simulink model "InverseDynamicsControlOperational"  (R2021b)
settings: Solver=VariableStepAuto  StartTime=0.0  StopTime=15  RelTol=1e-3
values from neighbouring files (symbols this model uses):
  F_v = zeros(6,6)    [param.m]
  K_d = 200.*eye(6,6)    [param.m]
  K_p = 1000.*eye(6,6)    [param.m]
undefined symbols (not defined in the file or in its folder): a, g, iner_l, pi_l, q_i
settings Model: Creator=ASUS  LastModifiedBy=ASUS

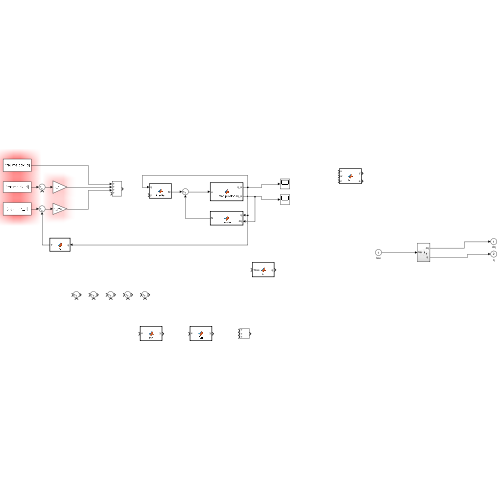
[thumbnail: Simulink's stored preview of the top-level diagram]
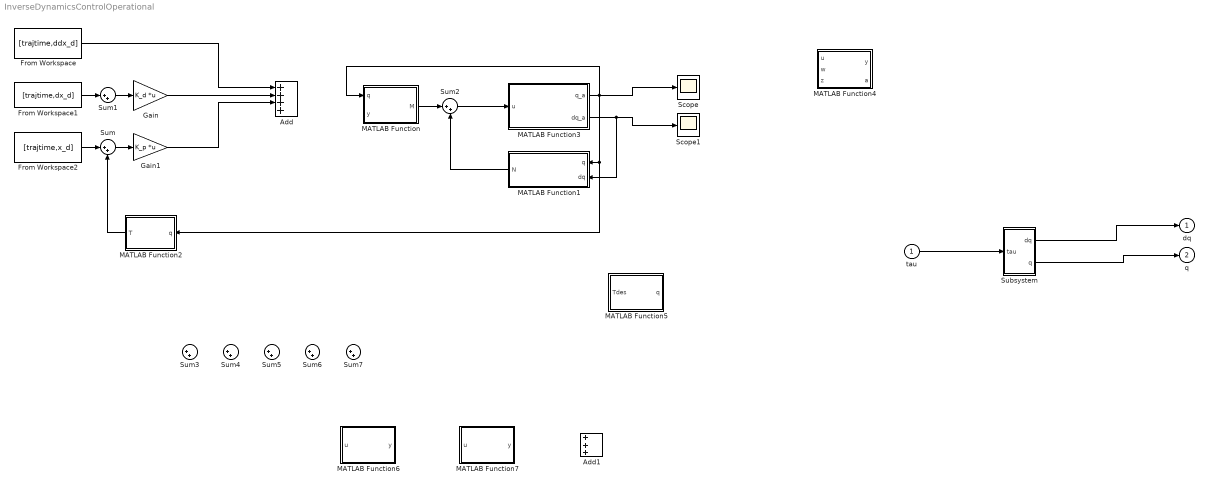
== system InverseDynamicsControlOperational ==
  tau : Inport
  Add : Sum  Inputs=++++
  Add1 : Sum  Inputs=+++
  From Workspace : FromWorkspace  VariableName=[trajtime,ddx_d]
  From Workspace1 : FromWorkspace  VariableName=[trajtime,dx_d]
  From Workspace2 : FromWorkspace  VariableName=[trajtime,x_d]
  Gain : Gain  Gain=K_d  Multiplication=Matrix(K*u)
  Gain1 : Gain  Gain=K_p  Multiplication=Matrix(K*u)
  MATLAB Function : MATLAB Function  TreatAsAtomicUnit=on
  MATLAB Function1 : MATLAB Function  TreatAsAtomicUnit=on
  MATLAB Function2 : MATLAB Function  TreatAsAtomicUnit=on
  MATLAB Function3 : MATLAB Function  TreatAsAtomicUnit=on
  MATLAB Function4 : MATLAB Function  TreatAsAtomicUnit=on
  MATLAB Function5 : MATLAB Function  TreatAsAtomicUnit=on
  MATLAB Function6 : MATLAB Function  TreatAsAtomicUnit=on
  MATLAB Function7 : MATLAB Function  TreatAsAtomicUnit=on
  Scope : Scope
  Scope1 : Scope
  Subsystem : Subsystem
  Sum{,1..7} (8 alike) : Sum  Inputs=|++
  dq : Outport  InitialOutput=0
  "q " : Outport  Port=2  InitialOutput=0
  wires:
  From Workspace/1 -> Add/1
  Gain/1 -> Add/2
  Gain1/1 -> Add/3
  From Workspace2/1 -> Sum/1
  Sum/1 -> Gain1/1
  From Workspace1/1 -> Sum1/1
  Sum1/1 -> Gain/1
  MATLAB Function2/1(T) -> Sum/2
  MATLAB Function/1(M) -> Sum2/1
  MATLAB Function1/1(N) -> Sum2/2
  Sum2/1 -> MATLAB Function3/1(u)
  MATLAB Function3/1(q_a) -> MATLAB Function/1(q), Scope/1, MATLAB Function2/1(q), MATLAB Function1/1(q)
  MATLAB Function3/2(dq_a) -> MATLAB Function1/2(dq), Scope1/1
  tau/1 -> Subsystem/1(tau)
  Subsystem/1(dq) -> dq/1
  Subsystem/2("q ") -> "q "/1

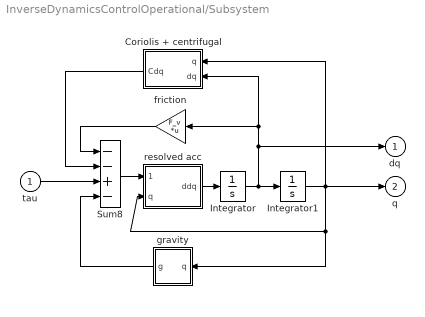
== system InverseDynamicsControlOperational/Subsystem ==
  tau : Inport
  Coriolis + centrifugal : Subsystem
      mask Display: disp('C(q,dq)dq')
  Integrator : Integrator  InitialCondition=[0 0]  ZeroCross=off
  Integrator1 : Integrator  InitialCondition=q_i  ZeroCross=off
  Sum8 : Sum  Inputs=--+-  InputSameDT=on  SaturateOnIntegerOverflow=on  OutDataTypeStr=Inherit: Same as first input
  friction : Gain  Gain=F_v  Multiplication=Matrix(K*u)  SaturateOnIntegerOverflow=on  OutDataTypeStr=Inherit: Same as input  ParamDataTypeStr=Inherit: Same as input
      mask Display: disp('F_v')
  gravity : Subsystem
      mask Display: disp('g(q)')
  resolved acc : Subsystem
      mask Display: disp('inv(B(q))')
  dq : Outport  InitialOutput=0
  "q " : Outport  Port=2  InitialOutput=0
  wires:
  Integrator/1 -> Integrator1/1, dq/1, Coriolis + centrifugal/2(dq), friction/1
  Integrator1/1 -> "q "/1, Coriolis + centrifugal/1(q), resolved acc/2(q), gravity/1(q)
  Sum8/1 -> resolved acc/1(tau-tau')
  gravity/1(g) -> Sum8/4
  tau/1 -> Sum8/3
  Coriolis + centrifugal/1(Cdq) -> Sum8/2
  friction/1 -> Sum8/1
  resolved acc/1(ddq) -> Integrator/1

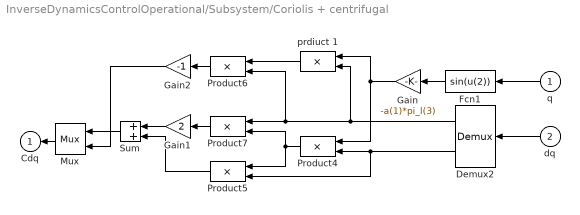
== system InverseDynamicsControlOperational/Subsystem/Coriolis + centrifugal ==
  q : Inport
  dq : Inport  Port=2
  Demux2 : Demux  Outputs=2
      settings: DisplayOption=none
  Fcn1 : Fcn  Expr=sin(u(2))
  Gain : Gain  Gain=-a(1)*pi_l(3)  SaturateOnIntegerOverflow=on  OutDataTypeStr=Inherit: Same as input  ParamDataTypeStr=Inherit: Same as input
      mask Display: disp('k_3')
  Gain1 : Gain  Gain=2  SaturateOnIntegerOverflow=on  OutDataTypeStr=Inherit: Same as input  ParamDataTypeStr=Inherit: Same as input
  Gain2 : Gain  Gain=-1  SaturateOnIntegerOverflow=on  OutDataTypeStr=Inherit: Same as input  ParamDataTypeStr=Inherit: Same as input
  Mux : Mux  Inputs=2
  Product{4..7} (4 alike) : Product  InputSameDT=on  RndMeth=Zero  SaturateOnIntegerOverflow=on  OutDataTypeStr=Inherit: Same as first input
  Sum : Sum  InputSameDT=on  SaturateOnIntegerOverflow=on  OutDataTypeStr=Inherit: Same as first input
  prdiuct 1 : Product  InputSameDT=on  RndMeth=Zero  SaturateOnIntegerOverflow=on  OutDataTypeStr=Inherit: Same as first input
  Cdq : Outport  InitialOutput=0
  wires:
  dq/1 -> Demux2/1
  Gain2/1 -> Mux/2
  Product6/1 -> Gain2/1
  Mux/1 -> Cdq/1
  Sum/1 -> Mux/1
  Product5/1 -> Sum/2
  Gain1/1 -> Sum/1
  Product7/1 -> Gain1/1
  Demux2/1 -> prdiuct 1/2, Product6/2, Product7/1
  Demux2/2 -> Product4/2, Product5/2
  prdiuct 1/1 -> Product6/1
  Gain/1 -> prdiuct 1/1, Product4/1
  Fcn1/1 -> Gain/1
  q/1 -> Fcn1/1
  Product4/1 -> Product5/1, Product7/2

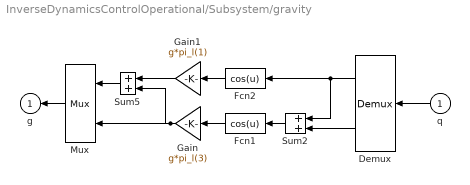
== system InverseDynamicsControlOperational/Subsystem/gravity ==
  q : Inport
  Demux : Demux  Outputs=2
      settings: DisplayOption=none
  Fcn1 : Fcn  Expr=cos(u)
  Fcn2 : Fcn  Expr=cos(u)
  Gain : Gain  Gain=g*pi_l(3)  SaturateOnIntegerOverflow=on  OutDataTypeStr=Inherit: Same as input  ParamDataTypeStr=Inherit: Same as input
      mask Display: disp('k_2')
  Gain1 : Gain  Gain=g*pi_l(1)  SaturateOnIntegerOverflow=on  OutDataTypeStr=Inherit: Same as input  ParamDataTypeStr=Inherit: Same as input
      mask Display: disp('k_1')
  Mux : Mux  Inputs=2
  Sum2 : Sum  InputSameDT=on  SaturateOnIntegerOverflow=on  OutDataTypeStr=Inherit: Same as first input
  Sum5 : Sum  InputSameDT=on  SaturateOnIntegerOverflow=on  OutDataTypeStr=Inherit: Same as first input
  g : Outport  InitialOutput=0
  wires:
  q/1 -> Demux/1
  Demux/2 -> Sum2/2
  Sum2/1 -> Fcn1/1
  Fcn1/1 -> Gain/1
  Fcn2/1 -> Gain1/1
  Demux/1 -> Fcn2/1, Sum2/1
  Gain1/1 -> Sum5/1
  Sum5/1 -> Mux/1
  Gain/1 -> Sum5/2, Mux/2
  Mux/1 -> g/1

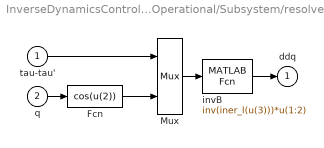
== system InverseDynamicsControlOperational/Subsystem/resolved acc ==
  tau-tau' : Inport
  q : Inport  Port=2
  Fcn : Fcn  Expr=cos(u(2))
  Mux : Mux  Inputs=[2,1]
  "invB " : MATLABFcn  MATLABFcn=inv(iner_l(u(3)))*u(1:2)  OutputDimensions=2
      mask Display: disp('inv(B(q))')
  ddq : Outport  InitialOutput=0
  wires:
  Fcn/1 -> Mux/2
  q/1 -> Fcn/1
  "invB "/1 -> ddq/1
  tau-tau'/1 -> Mux/1
  Mux/1 -> "invB "/1

== matlab function InverseDynamicsControlOperational/MATLAB Function1 ==
  data: q input; N output; dq input
function N = nonlin(q,dq)

% Extracting from input matrices
q1 = q(1);
q2 = q(2);
q3 = q(3);
q4 = q(4);
q5 = q(5);
q6 = q(6);

qd=dq;
qd1 = qd(1);
qd2 = qd(2);
qd3 = qd(3);
qd4 = qd(4);
qd5 = qd(5);
qd6 = qd(6);

global I1 I2 I3 I4 I5 I6 I7 I8 I9 I10 I11 I12 I13 I14 I15 I16 I17 I18 I19 I20 I21 I22 I23 Im g1 g2 g3 g4 g5

% Coriolis matrix elements
b112=2*(-I3*sin(q2)*cos(q2)+I5*cos(q2+q2+q3) +I7*sin(q2+q3)*cos(q2+q3) -I12*sin(q2+q2+q3)-I15*2*sin(q2+q3)*cos(q2+q3)+I16*cos(q2+q2+q3)+I21*sin(q2+q3)*cos(q2+q3)+I22*(1-2*sin(q2+q3)*sin(q2+q3)))+ I10*(1-sin(q2+q3)*sin(q2+q3))+I11*(1-2*sin(q2)*sin(q3));

b113=2*(I5*cos(q2)*cos(q2+q3)+I7*sin(q2+q3)*cos(q2+q3)-I12*cos(q2)*sin(q2+q2)+ I15*2*sin(q2+q3)*cos(q2+q3)+I16*cos(q2)*cos(q2+q3)+I21*sin(q2+q3)*cos(q2+q3)+I22*(1-2*sin(q2+q3)*sin(q2+q3)))+I10*(1-2*sin(q2+q3)*sin(q2+q3));

b115=2*(-sin(q2+q3)*cos(q2+q3)+I15*2*sin(q2+q3)*cos(q2+q3)+I16*cos(q2)*cos(q2+q3)+I22*cos(q2+q3)*cos(q2+q3));

b123=2*(-I8*sin(q2+q3)+I13*cos(q2+q3)+I18*sin(q2+q3));

b214=I14*sin(q2+q3)+I19*sin(q2+q3)+2*I20*sin(q2+q3)*(1-0.5);

b223=2*(-I12*sin(q3)+I5*cos(q3)+I16*cos(q3));

b225=2*(I16*cos(q3)+I21);

b235=2*(I16*cos(q3)+I22);

b314=2*(I20*sin(q2+q3)*(1-0.5))+I14*sin(q2+q3)+I19*sin(q2+q3);

b412=-1*(I14*sin(q2+q3)+I19*sin(q2+q3)+2*I20*sin(q2+q3)*(1-0.5));

b412=b214;

b413=-1*(I14*sin(q2+q3)+I19*sin(q2+q3)+2*I20*sin(q2+q3)*(1-0.5));

b413=-1*b314;

b415=-I20*sin(q2+q3)-I17*sin(q2+q3);

b514=I20*sin(q2+q3)+I17*sin(q2+q3);

% Coriolis Matrix B
B = zeros(15,6);

B(1,1) = b112;
B(1,2) = b113;
B(1,4) = b115;
B(1,6) = b123;

B(2,3) = b214;
B(2,6) = b223;
B(2,8) = b225;
B(2,11) = b235;

B(3,3) = b314;

B(4,1) = b412;
B(4,2) = b412;
B(4,4) = b415;

B(5,3) = b514;

% B_n = B.*[qd1*qd2; qd1*qd3; qd2*qd3; 0; 0; 0];

B_n = [b112*qd1*qd2 + b113*qd1*qd3 + b123*qd2*qd3;
    b223*qd2*qd3;
    0;
    b412*qd1*qd2 + b413*qd1*qd3;
    0;
    0];

% Centrifugal matrix elements
c12 = I4*cos(q2)-I8*sin(q2+q3)-I9*sin(q2)+I13*cos(q2+q3)+I18*sin(q2+q3);
c13 = 0.5*b123;
c21 = -0.5*b112;
c23 = 0.5*b223;
c31 = -0.5*b113;
c32 = -1*c23;

c51 = -0.5*b115;
c52 = -0.5*b225;

%Centrifugal matrix C
C=zeros(6,6);

C(1,2) = c12;
C(1,3) = c13;

C(2,1) = c21;
C(2,3) = c23;

C(3,1) = c31;
C(3,2) = c32;

C(5,1) = c51;
C(5,2) = c52;

% C_n = C.*[qd1^2; qd2^2; qd3^2; 0; 0; 0];

C_n = [c12*qd2^2 + c13*qd3^2;
    c21*qd1^2 + c23*qd3^2;
    c13*qd1^2 + c32*qd2^2;
    0;
    c51*qd1^2 + c52*qd2^2;
    0];

% Gravity matrix elements
G2 = (g1*cos(q1))+(g2*sin(q2+q3))+(g3*sin(q2))+(g4*cos(q2+q3))+(g5*sin(q2+q3));
G3 = (g2*sin(q2+q3))+(g4*cos(q2+q3))+(g5*sin(q2+q3));
G5 = g5*sin(q2+q3);

% Gravity matrix G

G_n = [0; G2; G3; 0; G5; 0];

N = B_n + C_n + G_n;

end

== matlab function InverseDynamicsControlOperational/MATLAB Function ==
  data: q input; M output; y input
function M = inertia(q,y)

% Extracting from input matrix
q1 = q(1);
q2 = q(2);
q3 = q(3);
q4 = q(4);
q5 = q(5);
q6 = q(6);

% Intertial constant reference (Kg.m^2)
global I1 I2 I3 I4 I5 I6 I7 I8 I9 I10 I11 I12 I13 I14 I15 I16 I17 I18 I19 I20 I21 I22 I23 Im g1 g2 g3 g4 g5

% Inertia matrix elements
M11 = Im(1)+I1+(I3*cos(q2)*cos(q2))+(I7*sin(q2+q3)*sin(q2+q3))+(I10*sin(q2+q3)*cos(q2+q3))+(I11*sin(q2)*cos(q2))+(I21*sin(q2+q3)*sin(q2+q3))+2+(I5*cos(q2)*sin(q2+q3))+(I12*cos(q2)*cos(q2+q3))+(I15*sin(q2+q3)*sin(q2+q3))+(I16*cos(q2)*sin(q2+q3))+(I22*sin(q2+q3)*cos(q2+q3));

M12 = (I4*sin(q2))+(I8*cos(q2+q3))+(I9*cos(q2))+(I13*sin(q2+q3))-(I18*cos(q2+q3));

M13 = (I8*cos(q2+q3))+(I13*sin(q2+q3))-(I18*cos(q2+q3));

M22 = Im(2)+I2+I6+2*(I5*sin(q3)+I12*cos(q2)+I15+I16*sin(q3));

M23 = (I5*sin(q3))+I6+(I12*cos(q3))+(I16*sin(q3))+(2*I15);

M33 = Im(3)+I6+(2*I15);

M35 = I15+I17;

M44 = Im(4)+I14;

M55 = Im(5)+I17;

M66 = Im(6)+I23;

M21 = M12;

M31 = M13;

M32 = M23;

%% M Matrix with coupling interactions- Centralized Control

M = [M11 M12 M13 0 0 0;
    M21 M22 M23 0 0 0;
    M31 M32 M33 0 M35 0;
    0 0 0 M44 0 0;
    0 0 0 0 M55 0;
    0 0 0 0 0 M66];

end

== matlab function InverseDynamicsControlOperational/MATLAB Function2 ==
  data: q input; T output
function T = fk(q)

% Extracting from input matrix
q1 = q(1);
q2 = q(2);
q3 = q(3);
q4 = q(4);
q5 = q(5);
q6 = q(6);

%Robot Definition
global a2 a3 a6 d2 d3 d4

L1 = Link('revolute','d', 0, 'a', 0,'alpha', 0, 'modified', 'qlim',[-2*pi,2*pi]);
L2 = Link('revolute','d', d2, 'a', 0,'alpha', -pi/2, 'modified', 'qlim',[-2*pi,2*pi]);
L3 = Link('revolute','d', d3, 'a', a2,'alpha', 0, 'modified', 'qlim',[-2*pi,2*pi]);
L4 = Link('revolute','d', d4, 'a', a3,'alpha', pi/2, 'modified', 'qlim',[-2*pi,2*pi]);
L5 = Link('revolute','d', 0, 'a', 0,'alpha', -pi/2, 'modified', 'qlim',[-2*pi,2*pi]);
L6 = Link('revolute','d', 0, 'a', 0,'alpha', pi/2, 'modified', 'qlim',[-2*pi,2*pi]);

Puma560 = SerialLink([L1 L2 L3 L4 L5 L6],'name','Puma560');
DH_Mod=[q1 q2 q3 q4 q5 q6];

Tdes = vpa(simplify(Puma560.fkine(DH_Mod)),5);

T = [Tdes.n Tdes.o Tdes.a Tdes.t;
    0 0 0 1];

end

== matlab function InverseDynamicsControlOperational/MATLAB Function3 ==
  data: u input; q_a output; dq_a output
function [q_a,dq_a] = manipulator(u)
q_a=0;
dq_a=0;
end

== matlab function InverseDynamicsControlOperational/MATLAB Function4 ==
  data: u input; y output; w input; z input; a output
function [y,a] = fcn(u,w,z)
%#codegen

y = u;
a=y;

== matlab function InverseDynamicsControlOperational/MATLAB Function5 ==
  data: Tdes input; q output
%% Inverse Kinematics

function q = ik(Tdes)

%Robot Definition
% a2 = 0.4318; a3 = 0.0191; a6 = 0.1;
% d3 = 0.1254; d4 = 0.4318;


% a2 = 0.4318; a3 = -0.0203; a6 = 0.1;
% d2=0.2435; d3 = -0.0934; %d3 = 0.1254; 
% d4 = 0.4331;
global a2 a3 a6 d2 d3 d4

%Definining Tdes
% x = Tdes(1,4); y = Tdes(2,4); z = Tdes(3,4);
% r11 = Tdes(1,1); r21 = Tdes(2,1); r31 = Tdes(3,1);
% r12 = Tdes(1,2); r22 = Tdes(2,2); r32 = Tdes(3,2);
% r13 = Tdes(1,3); r23 = Tdes(2,3); r33 = Tdes(3,3);
% 
% t1 = atan2(y,x) - atan2(d3, +1*sqrt(x^2 + y^2 - d3^2)); %Joint 1
% 
% K = (x^2 + y^2 + z^2 - a2^2 - a3^2 - d3^2 - d4^2)/(2*a2);
% 
% t3 = atan2(a3,d4) - atan2(K, 1*sqrt(a3^2 + d4^2 - K^2)); %Joint 3
% 
% t23 = atan2((-a3-a2*cos(t3))*z - (cos(t1)*x+sin(t1)*y)*(d4-a2*sin(t3)), z*(a2*sin(t3)-d4) + (a3+a2*cos(t3))*(cos(t1)*x+sin(t1)*y));
% 
% t2 = t23 - t3; %Joint 2
% 
% s4 = -r13*sin(t1) + r23*cos(t1);
% c4 = -r13*cos(t1)*cos(t23) - r23*sin(t1)*cos(t23) + r33*sin(t23);
% t4 = atan2(s4, c4); %Joint 4
% 
% s5 = -r13*(cos(t1)*cos(t23)*cos(t4)+sin(t1)*sin(t4)) - r23*(sin(t1)*cos(t23)*cos(t4)-cos(t1)*sin(t4)) + r33*sin(t23)*cos(t4);
% c5 = -r13*cos(t1)*sin(t23) - r23*sin(t1)*sin(t23) - r33*cos(t23);
% t5 = atan2(s5, c5); %Joint 5
% 
% s6 = -r11*(cos(t1)*cos(t23)*sin(t4) - sin(t1)*cos(t4)) - r21*(sin(t1)*cos(t23)*sin(t4) + cos(t1)*cos(t4)) + r31*sin(t23)*sin(t4);
% c6 = r11*(cos(t5)*(cos(t1)*cos(t4)*cos(t23)+sin(t1)*sin(t4)) - cos(t1)*sin(t5)*sin(t23)) + r21*(cos(t5)*(sin(t1)*cos(t4)*cos(t23) - cos(t1)*sin(t4)) - sin(t1)*sin(t5)*sin(t23)) - r31*(sin(t5)*cos(t23) + cos(t4)*cos(t5)*sin(t23));
% t6 = atan2(s6, c6); %Joint 6
% 
% Puma560_IK = [t1,t2,t3,t4,t5,t6];

L1 = Link('revolute','d', 0, 'a', 0,'alpha', 0, 'modified', 'qlim',[-2*pi,2*pi]);
L2 = Link('revolute','d', d2, 'a', 0,'alpha', -pi/2, 'modified', 'qlim',[-2*pi,2*pi]);
L3 = Link('revolute','d', d3, 'a', a2,'alpha', 0, 'modified', 'qlim',[-2*pi,2*pi]);
L4 = Link('revolute','d', d4, 'a', a3,'alpha', pi/2, 'modified', 'qlim',[-2*pi,2*pi]);
L5 = Link('revolute','d', 0, 'a', 0,'alpha', -pi/2, 'modified', 'qlim',[-2*pi,2*pi]);
L6 = Link('revolute','d', 0, 'a', 0,'alpha', pi/2, 'modified', 'qlim',[-2*pi,2*pi]);

p560 = SerialLink([L1 L2 L3 L4 L5 L6],'name','Puma560');

q = p560.ikine(Tdes)

%p560.plot(q)

end

== matlab function InverseDynamicsControlOperational/MATLAB Function6 ==
  data: u input; y output
function y = fcn(u)

y = u;

== matlab function InverseDynamicsControlOperational/MATLAB Function7 ==
  data: u input; y output
function y = fcn(u)

y = u;
